simulink library "atlas_impctrl_library"  (Simulink 8.5)
settings: Solver=ode45  StartTime=0.0  StopTime=10.0  RelTol=1e-3
values from neighbouring files (symbols this model uses):
  B = d - 0.1*ones(NJL,1)    [atlas_joint_impctrl_sqrt_damping_test_settings_default.m]
  D = 0.7*eye(NJL)    [atlas_joint_impctrl_sqrt_damping_test_settings_default.m]
  K_d = 150*eye(NJL)    [atlas_joint_impctrl_sqrt_damping_test_settings_default.m]
  K_ext_c = 0    [atlas_joint_impctrl_sqrt_damping_test_settings_default.m]
  K_ext_o = 1    [atlas_joint_impctrl_sqrt_damping_test_settings_default.m]
  K_fri_o = 1    [atlas_joint_impctrl_sqrt_damping_test_settings_default.m]
  K_O = 5*eye(NJL)    [atlas_joint_impctrl_sqrt_damping_test_settings_default.m]
  K_obs_c = 0    [atlas_joint_impctrl_sqrt_damping_test_settings_default.m]
  K_qD_d = 1    [atlas_joint_impctrl_sqrt_damping_test_settings_default.m]
  K_qDD_d = 1    [atlas_joint_impctrl_sqrt_damping_test_settings_default.m]
  K_tau_a = 1    [atlas_joint_impctrl_sqrt_damping_test_settings_default.m]
  K_tau_c = 1    [atlas_joint_impctrl_sqrt_damping_test_settings_default.m]
  K_tau_D = 1    [atlas_joint_impctrl_sqrt_damping_test_settings_default.m]
  K_tau_e = 0    [atlas_joint_impctrl_sqrt_damping_test_settings_default.m]
  K_tau_f = 0    [atlas_joint_impctrl_sqrt_damping_test_settings_default.m]
  K_tau_g = 1    [atlas_joint_impctrl_sqrt_damping_test_settings_default.m]
  K_tau_K = 1    [atlas_joint_impctrl_sqrt_damping_test_settings_default.m]
  K_tau_o = 0    [atlas_joint_impctrl_sqrt_damping_test_settings_default.m]
  qD_th = 0.05*ones(NJL,1)    [atlas_joint_impctrl_sqrt_damping_test_settings_default.m]
  T = 0.001    [atlas_joint_impctrl_sqrt_damping_test_settings_default.m]
  T1 = 0    [atlas_joint_impctrl_sqrt_damping_test_settings_default.m]
  tau_c = muC - 4*ones(NJL,1)    [atlas_joint_impctrl_sqrt_damping_test_settings_default.m]
  tau_th = 0.02*ones(NJL,1)    [atlas_joint_impctrl_sqrt_damping_test_settings_default.m]
undefined symbols (not defined in the file or in its folder): K_tau_F, mr, offsets
undefined symbols (not defined in the file): atlas_arm_lr, atlas_leg_lr, delta_s, MPV, MPV_arm_damp, MPV_arm_model, MPV_leg_damp, MPV_leg_model, qD_s, tau_s
libraries: atlas_dynamic_library x23, atlas_impctrl_library x18, dspmtrx3 x3
(part 2 of 2)

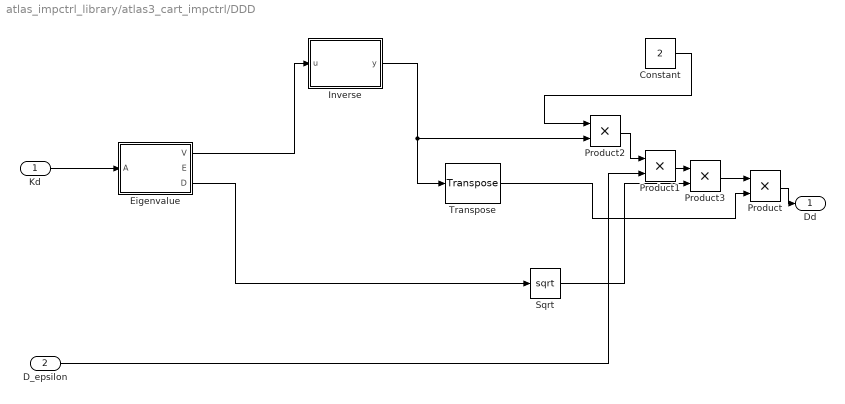
== system atlas_impctrl_library/atlas3_cart_impctrl/DDD ==
  Kd : Inport
  D_epsilon : Inport  Port=2
  Constant : Constant  Value=2
  Eigenvalue : MATLAB Function  TreatAsAtomicUnit=on
  Inverse : MATLAB Function  TreatAsAtomicUnit=on
  Product{,1..3} (4 alike) : Product
  Sqrt : Sqrt  SaturateOnIntegerOverflow=on
  Transpose : dspmtrx3/Transpose  Hermitian=off  overflowFlag=off
  Dd : Outport
  wires:
  Kd/1 -> Eigenvalue/1(A)
  Eigenvalue/1(V) -> Inverse/1(u)
  Inverse/1(y) -> Product2/2, Transpose/1
  Eigenvalue/3(D) -> Sqrt/1
  Product/1 -> Dd/1
  Constant/1 -> Product2/1
  Product2/1 -> Product1/1
  Product1/1 -> Product3/1
  Product3/1 -> Product/1
  Sqrt/1 -> Product3/2
  Transpose/1 -> Product/2
  D_epsilon/1 -> Product1/2

== system atlas_impctrl_library/atlas3_cart_impctrl/lambda ==
  M : Inport
  J-T : Inport  Port=2
  J-1 : Inport  Port=3
  Product3 : Product
  produkt : Product
  Lambda : Outport
  wires:
  M/1 -> Product3/2
  J-1/1 -> produkt/2
  produkt/1 -> Lambda/1
  Product3/1 -> produkt/1
  J-T/1 -> Product3/1

== system atlas_impctrl_library/atlas3_cart_impctrl/mu ==
  M : Inport
  J-1 : Inport  Port=2
  JD : Inport  Port=3
  JDT : Inport  Port=4
  tauC : Inport  Port=5
  Product5 : Product
  Product6 : Product
  Product7 : Product
  Sum3 : Sum  Inputs=|+-
  mu : Product
  mu(x,xD) : Outport
  wires:
  JDT/1 -> Product5/1
  M/1 -> Product7/1
  Product5/1 -> mu/1
  mu/1 -> mu(x,xD)/1
  tauC/1 -> Sum3/1
  Product7/1 -> Product6/1
  Product6/1 -> Sum3/2
  Sum3/1 -> Product5/2
  J-1/1 -> mu/2, Product7/2
  JD/1 -> Product6/2

== system atlas_impctrl_library/atlas3_cart_impctrl/xD und xDD ==
  J : Inport
  qD : Inport  Port=2
  qDD : Inport  Port=3
  JD : Inport  Port=4
  Product : Product
  Product2 : Product
  Sum1 : Sum  Inputs=|++
  iwas : Product
  XDD : Outport
  xD : Outport  Port=2
  wires:
  JD/1 -> Product2/1
  J/1 -> Product/1, iwas/1
  Product/1 -> Sum1/1
  qDD/1 -> Product/2
  Sum1/1 -> XDD/1
  qD/1 -> Product2/2, iwas/2
  iwas/1 -> xD/1
  Product2/1 -> Sum1/2

== matlab function double_diag/MATLAB double_diag ==
  data: M input double; K_d parameter double; D_d output double; D parameter double
function D_d=double_diag(M,K_d,D)
%#codegen
[V,K0]=eig(K_d,M);
% Q=inv(V)';
% D_d_=2*Q*D*sqrt(K0)*Q';
QD=V'\D;
Y=2*QD*sqrt(K0);
D_d_=Y/V;
assert(max(max(abs(imag(D_d_))))==0);
D_d=real(D_d_);

== matlab function atlas3_cart_impctrl/DDD/Eigenvalue ==
  data: A input double; V output double; E output double; D output double
function [V,E,D] = fcn(A)

E=eig(A);
[V,D]=eig(A);

== matlab function sqrt_damping/MATLAB sqrt_damping ==
  data: M input double; K_d parameter double; D_d output double; D parameter double
function D_d=sqrt_damping(M,K_d,D)
%#codegen
K_d1=sqrtm(K_d);
M1=sqrtm(M);
D_d_=K_d1*D*M1+M1*D*K_d1;
assert(max(max(abs(imag(D_d_))))==0);
D_d=real(D_d_);

== matlab function atlas3_cart_impctrl/MATLAB J ==
  data: qs input double; Jg output double
function Jg = fcn(qs)

lr = true;

Jg = atlas3_arm_jacobig_sym(qs, lr);

== matlab function atlas3_cart_impctrl/MATLAB JD ==
  data: u input double; y output double
function y = fcn(u)
%#codegen

y = u;

== matlab function atlas3_cart_impctrl/DDD/Inverse ==
  data: u input double; y output double
function y = fcn(u)
%#codegen

y = inv(u);

== matlab function atlas3_cart_impctrl/Inverse ==
  data: u input double; y output double
function y = fcn(u)
%#codegen

y = u;

== matlab function friction_compensation/MATLAB sqrt_damping ==
  data: tau_imp input double; qD input double; tau_F output double; tau_c parameter double; B parameter double; qD_th parameter double; tau_th parameter double
function tau_F=sqrt_damping(tau_imp,qD,tau_c,B,qD_th,tau_th)
%#codegen
tau_F=zeros(length(tau_imp),1);
for i=1:length(tau_imp)
  % friction compensation only, when significant distance to desired
  % trajectory
  if (abs(tau_imp(i)) > tau_th(i))
    % when qD<qD_th stiction is assumed and even if speed is in opposite
    % direction, full compensation force is applied, this is to avoid
    % sensor noise induced jitter
    if (abs(qD(i)) > qD_th(i) || sign(qD(i))==sign(tau_imp(i)))
      tau_F(i) = tau_c(i)*sign(qD(i)) + B(i)*qD(i);
    else
      tau_F(i) = tau_c(i);
    end
  else
    tau_F(i) = 0;
  end
end

== matlab function velocity_based_friction_observer/MATLAB Function ==
  data: tau_J_old input double; tau_fr output double; tau_g_old input double; tau_c_old input double; tau_fr_old input double; tau_int_alt input double; qD input double; M input double; K_O parameter double; T parameter double; tau_int output double
function [tau_fr, tau_int] = fcn(tau_J_old, tau_g_old, tau_c_old, tau_fr_old, tau_int_alt, qD, M, K_O, T)
%#codegen

tau_int = tau_int_alt + T*K_O*(M\(tau_J_old-tau_g_old-tau_c_old-tau_fr_old));
tau_fr  = tau_int - K_O*qD;

== matlab function compensate_hand_mass_and_offset/compensate_hand_mass_and_offset ==
  data: W_raw input double; W_comp output double; g_hand input double; mr parameter double; offsets parameter double
function W_comp = fcn(W_raw, g_hand, mr, offsets)
%#codegen

% mr contains the mass (1) and the coordinates of the com (2-4) of the hand
% (in hand coordinates), g has to be expressed in hand coordinates
W_comp = W_raw - offsets;
W_comp(1:3) = W_comp(1:3) - mr(1)*g;
W_comp(4:6) = W_comp(4:6) - cross(mr(2:4), mr(1)*g);

== matlab function momentum_based_friction_observer/MATLAB Function ==
  data: tau_J_old input double; tau_fr output double; tau_g_old input double; tau_c_old input double; tau_ext_old input double; tau_fr_obs_old input double; tau_int_old input double; qD input double; qD_old input double; M input double; M_old input double; MD_old input double; tau_fr_model_old input double; K_O parameter double; T1 parameter double size=[1 1]; tau_out_max parameter double; T parameter double size=[1 1]; tau_int output double; MD output double
function [tau_fr, tau_int, MD] = fcn(tau_J_old, tau_g_old, tau_c_old, tau_ext_old, tau_fr_obs_old, tau_int_old, qD, qD_old, M, M_old, MD_old, tau_fr_model_old, K_O, T1, tau_out_max, T)
%#codegen

MD      = 1/(T1+T) * (T1*MD_old + M - M_old);
tau_int = tau_int_old + T*(tau_J_old-tau_g_old-tau_c_old+tau_ext_old-tau_fr_model_old+MD*qD_old-tau_fr_obs_old);
tau_fr_MqD = -K_O*M*qD;
tau_fr = K_O*tau_int + tau_fr_MqD;

% limit output and anti-windup
for i=1:length(tau_J_old)
  if tau_fr(i)>tau_out_max(i)
    tau_fr(i)=tau_out_max(i);
    tau_int(i)=1/K_O(i,i)*(tau_out_max(i)-tau_fr_MqD(i));
  elseif tau_fr(i)<-tau_out_max(i)
    tau_fr(i)=-tau_out_max(i);
    tau_int(i)=1/K_O(i,i)*(-tau_out_max(i)-tau_fr_MqD(i));
  end
end

== matlab function fr_comp_w_obs/MATLAB fr_comp_w_obs ==
  data: tau_imp input double; qD input double; tau_F output double; tau_fr_model input double; tau_c parameter double; qD_th parameter double; tau_th parameter double
function tau_F=fr_comp_w_obs(tau_imp,qD,tau_fr_model,tau_c,qD_th,tau_th)
%#codegen
tau_F=zeros(length(tau_imp),1);
for i=1:length(tau_imp)
  if (abs(qD(i)) > qD_th(i))
    tau_F(i) = tau_fr_model(i);
  else
    % for low speed friction compensation only, when significant distance
    % to desired trajectory
    if (abs(tau_imp(i)) > tau_th(i))
      % when qD<qD_th stiction is assumed and even if speed is in opposite
      % direction, full compensation force is applied, this is to avoid
      % sensor noise induced jitter
      if (sign(qD(i))==sign(tau_imp(i)))
        tau_F(i) = tau_fr_model(i);
      else
        tau_F(i) = tau_c(i);
      end
    else
      tau_F(i) = 0;
    end
  end
end

== matlab function atlas_friction_model_atan/atlas_friction_model_atan ==
  data: qD input double; tau_fr_model output double; tau_c parameter double; B parameter double
function tau_fr_model = fcn(qD, tau_c, B)
%#codegen
tau_fr_model=zeros(length(qD),1);
for i=1:length(qD)
  tau_fr_model(i)=tau_c(i)*2/pi*atan(100*qD(i)) + B(i)*qD(i);
end

== matlab function atlas_friction_model/atlas_friction_model ==
  data: qD input double; tau_fr_model output double; tau_c parameter double; B parameter double
function tau_fr_model = fcn(qD, tau_c, B)
%#codegen
tau_fr_model=zeros(length(qD),1);
for i=1:length(qD)
  tau_fr_model(i)=tau_c(i)*sign(qD(i)) + B(i)*qD(i);
end
